simulink model "pneumatic_tank"  (R2018b)
settings: Solver=ode15s  StartTime=0.0  StopTime=30  FixedStep=1e-3  RelTol=1e-3
PreLoadFcn:
  | delta_p = 0.6; % MPa
  | p_init = 0.101325; % MPa
  | T_init = 293.15; % K
  | T_atm = 293.15; % K
  | 
  | A_valve_max = 4e-6; % m^2
  | A_valve_min = 1e-10; % m^2
  | 
  | A_pipe = 5e-6; % m^2
  | L_pipe = 1; % m
  | 
  | A_piston = 0.002; % m^2
  | L_piston = 0.2; % m
libraries: fl_lib x31, nesl_utility x6
(part 3 of 3)

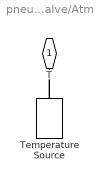
== system pneumatic_tank/Tank and valve/Atm ==
  Temperature Source : fl_lib/Thermal/Thermal Sources/Temperature Source  temperature=T_atm K
      settings: SourceProductName=Simscape
  T : PMIOPort  Side=Right
  connections:
  Temperature Source/LConn1 -- T/RConn1

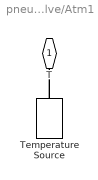
== system pneumatic_tank/Tank and valve/Atm1 ==
  Temperature Source : fl_lib/Thermal/Thermal Sources/Temperature Source  temperature=T_atm K
      settings: SourceProductName=Simscape
  T : PMIOPort  Side=Right
  connections:
  Temperature Source/LConn1 -- T/RConn1

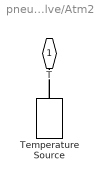
== system pneumatic_tank/Tank and valve/Atm2 ==
  Temperature Source : fl_lib/Thermal/Thermal Sources/Temperature Source  temperature=T_atm K
      settings: SourceProductName=Simscape
  T : PMIOPort  Side=Right
  connections:
  Temperature Source/LConn1 -- T/RConn1

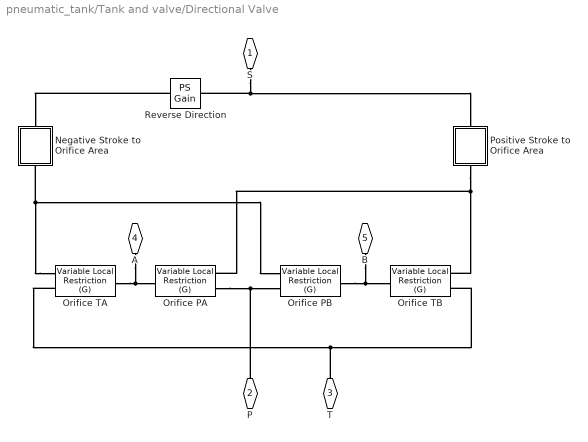
== system pneumatic_tank/Tank and valve/Directional Valve ==
  Negative Stroke to Orifice Area : Subsystem
  Orifice PA : fl_lib/Gas/Elements/Variable Local Restriction (G)  min_area=A_leakage m^2  max_area=A_max m^2  area=A_port m^2  Cd=Cd  B_lam=0.999  mdot_A_specify=off  mdot_A_priority=None  mdot_A=1e-6 kg/s  mdot_A_nominal_specify=off  mdot_A_nominal_unit=kg/s  mdot_A_nominal_value=1
      settings: SourceProductName=Simscape  SourceProductBaseCode=SS
  Orifice PB : fl_lib/Gas/Elements/Variable Local Restriction (G)  min_area=A_leakage m^2  max_area=A_max m^2  area=A_port m^2  Cd=Cd  B_lam=0.999  mdot_A_specify=off  mdot_A_priority=None  mdot_A=1e-6 kg/s  mdot_A_nominal_specify=off  mdot_A_nominal_unit=kg/s  mdot_A_nominal_value=1
      settings: SourceProductName=Simscape  SourceProductBaseCode=SS
  Orifice TA : fl_lib/Gas/Elements/Variable Local Restriction (G)  min_area=A_leakage m^2  max_area=A_max m^2  area=A_port m^2  Cd=Cd  B_lam=0.999  mdot_A_specify=off  mdot_A_priority=None  mdot_A=1e-6 kg/s  mdot_A_nominal_specify=off  mdot_A_nominal_unit=kg/s  mdot_A_nominal_value=1
      settings: SourceProductName=Simscape  SourceProductBaseCode=SS
  Orifice TB : fl_lib/Gas/Elements/Variable Local Restriction (G)  min_area=A_leakage m^2  max_area=A_max m^2  area=A_port m^2  Cd=Cd  B_lam=0.999  mdot_A_specify=off  mdot_A_priority=None  mdot_A=1e-6 kg/s  mdot_A_nominal_specify=off  mdot_A_nominal_unit=kg/s  mdot_A_nominal_value=1
      settings: SourceProductName=Simscape  SourceProductBaseCode=SS
  Positive Stroke to Orifice Area : Subsystem
  Reverse Direction : fl_lib/Physical Signals/Functions/PS Gain  gain=-1
  S : PMIOPort  Side=Left
  P : PMIOPort  Port=2  Side=Left
  T : PMIOPort  Port=3  Side=Left
  A : PMIOPort  Port=4  Side=Right
  B : PMIOPort  Port=5  Side=Right
  connections:
  Orifice PB/RConn1 -- B/RConn1 -- Orifice TB/RConn1
  Orifice TA/RConn1 -- Orifice PA/RConn1 -- A/RConn1
  Orifice TA/LConn1 -- T/RConn1 -- Orifice TB/LConn1
  Orifice PA/LConn1 -- P/RConn1 -- Orifice PB/LConn1
  S/RConn1 -- Positive Stroke to Orifice Area/LConn1 -- Reverse Direction/LConn1
  Positive Stroke to Orifice Area/RConn1 -- Orifice TB/LConn2 -- Orifice PA/LConn2
  Orifice TA/LConn2 -- Negative Stroke to Orifice Area/RConn1 -- Orifice PB/LConn2
  Reverse Direction/RConn1 -- Negative Stroke to Orifice Area/LConn1

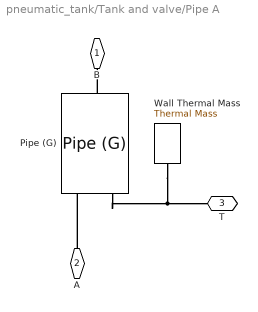
== system pneumatic_tank/Tank and valve/Pipe A ==
  Pipe (G) : fl_lib/Gas/Elements/Pipe (G)  length=L_pipe m  area=A_pipe m^2  Dh=2*sqrt(A_pipe/pi) m  length_add=0.1 * L_pipe m  roughness=15e-6 m  Re_lam=2000  Re_tur=4000  shape_factor=64  Nu_lam=3.66  p_pipe_specify=on  p_pipe_priority=High  p_pipe=p_init bar  p_pipe_nominal_specify=off  p_pipe_nominal_unit=MPa  p_pipe_nominal_value=1  T_pipe_specify=on  T_pipe_priority=High  T_pipe=T_init K  T_pipe_nominal_specify=off  T_pipe_nominal_unit=K  T_pipe_nominal_value=1  rho_pipe_specify=off  rho_pipe_priority=None  rho_pipe=1.2 kg/m^3  rho_pipe_nominal_specify=off  rho_pipe_nominal_unit=kg/m^3  rho_pipe_nominal_value=1
      settings: SourceProductName=Simscape  SourceProductBaseCode=SS
  Wall Thermal Mass : fl_lib/Thermal/Thermal Elements/Thermal Mass  mass=rho_wall * A_pipe * L_pipe kg  sp_heat=cp_wall J/kg/K  T_specify=on  T_priority=High  T=T_init K  T_nominal_specify=off  T_nominal_unit=K  T_nominal_value=1  Q_specify=off  Q_priority=None  Q=0 W  Q_nominal_specify=off  Q_nominal_unit=W  Q_nominal_value=1
  B : PMIOPort  Side=Right
  A : PMIOPort  Port=2  Side=Left
  T : PMIOPort  Port=3  Side=Left
  connections:
  Pipe (G)/RConn1 -- B/RConn1
  A/RConn1 -- Pipe (G)/LConn1
  Pipe (G)/LConn2 -- Wall Thermal Mass/LConn1 -- T/RConn1

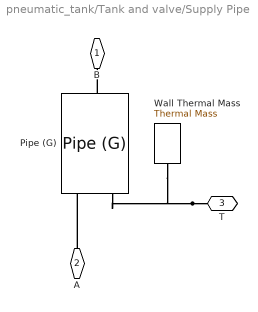
== system pneumatic_tank/Tank and valve/Supply Pipe ==
  Pipe (G) : fl_lib/Gas/Elements/Pipe (G)  length=L_pipe m  area=A_pipe m^2  Dh=2*sqrt(A_pipe/pi) m  length_add=0.1 * L_pipe m  roughness=15e-6 m  Re_lam=2000  Re_tur=4000  shape_factor=64  Nu_lam=3.66  p_pipe_specify=on  p_pipe_priority=High  p_pipe=p_init bar  p_pipe_nominal_specify=off  p_pipe_nominal_unit=MPa  p_pipe_nominal_value=1  T_pipe_specify=on  T_pipe_priority=High  T_pipe=T_init K  T_pipe_nominal_specify=off  T_pipe_nominal_unit=K  T_pipe_nominal_value=1  rho_pipe_specify=off  rho_pipe_priority=None  rho_pipe=1.2 kg/m^3  rho_pipe_nominal_specify=off  rho_pipe_nominal_unit=kg/m^3  rho_pipe_nominal_value=1
      settings: SourceProductName=Simscape  SourceProductBaseCode=SS
  Wall Thermal Mass : fl_lib/Thermal/Thermal Elements/Thermal Mass  mass=rho_wall * A_pipe * L_pipe kg  sp_heat=cp_wall J/kg/K  T_specify=on  T_priority=High  T=T_init K  T_nominal_specify=off  T_nominal_unit=K  T_nominal_value=1  Q_specify=off  Q_priority=None  Q=0 W  Q_nominal_specify=off  Q_nominal_unit=W  Q_nominal_value=1
  B : PMIOPort  Side=Right
  A : PMIOPort  Port=2  Side=Left
  T : PMIOPort  Port=3  Side=Left
  connections:
  T/RConn1 -- Wall Thermal Mass/LConn1 -- Pipe (G)/LConn2
  A/RConn1 -- Pipe (G)/LConn1
  Pipe (G)/RConn1 -- B/RConn1

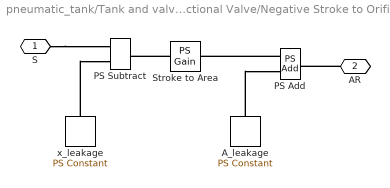
== system pneumatic_tank/Tank and valve/Directional Valve/Negative Stroke to Orifice Area ==
  A_leakage : fl_lib/Physical Signals/Sources/PS Constant  constant=A_leakage
  PS Add : fl_lib/Physical Signals/Functions/PS Add
  PS Subtract : fl_lib/Physical Signals/Functions/PS Subtract
      settings: SourceProductName=Simscape
  Stroke to Area : fl_lib/Physical Signals/Functions/PS Gain  gain=(A_max - A_leakage) / (x_max - x_leakage)
  x_leakage : fl_lib/Physical Signals/Sources/PS Constant  constant=x_leakage
  S : PMIOPort  Side=Left
  AR : PMIOPort  Port=2  Side=Right
  connections:
  S/RConn1 -- PS Subtract/LConn1
  PS Add/LConn1 -- Stroke to Area/RConn1
  Stroke to Area/LConn1 -- PS Subtract/RConn1
  A_leakage/RConn1 -- PS Add/LConn2
  x_leakage/RConn1 -- PS Subtract/LConn2
  AR/RConn1 -- PS Add/RConn1

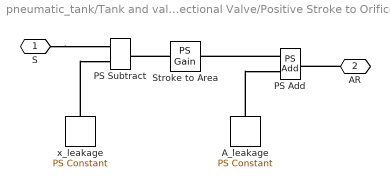
== system pneumatic_tank/Tank and valve/Directional Valve/Positive Stroke to Orifice Area ==
  A_leakage : fl_lib/Physical Signals/Sources/PS Constant  constant=A_leakage
  PS Add : fl_lib/Physical Signals/Functions/PS Add
  PS Subtract : fl_lib/Physical Signals/Functions/PS Subtract
      settings: SourceProductName=Simscape
  Stroke to Area : fl_lib/Physical Signals/Functions/PS Gain  gain=(A_max - A_leakage) / (x_max - x_leakage)
  x_leakage : fl_lib/Physical Signals/Sources/PS Constant  constant=x_leakage
  S : PMIOPort  Side=Left
  AR : PMIOPort  Port=2  Side=Right
  connections:
  AR/RConn1 -- PS Add/RConn1
  x_leakage/RConn1 -- PS Subtract/LConn2
  A_leakage/RConn1 -- PS Add/LConn2
  Stroke to Area/LConn1 -- PS Subtract/RConn1
  PS Add/LConn1 -- Stroke to Area/RConn1
  S/RConn1 -- PS Subtract/LConn1
